simulink model "DaoBaoTin_20151230_Cau2e"  (R2018a)
settings: Solver=FixedStepAuto  StartTime=0.0  StopTime=4  FixedStep=0.01  RelTol=1e-3
values from neighbouring files (symbols this model uses):
  A = [0 1; -0.1 -0.1]    [DaoBaoTin_20151230_Cau1d.m]    (also in DaoBaoTin_20151230_Cau2d.m = [-8.3164 0.0358; -0.7814 -4.0012])
  B = [0.1; 0.09]    [DaoBaoTin_20151230_Cau1d.m]    (also in DaoBaoTin_20151230_Cau2d.m = [0; 2])
  C = [1 0; 0 1]    [DaoBaoTin_20151230_Cau1d.m]    (also in DaoBaoTin_20151230_Cau2d.m)
  D = [0; 0]    [DaoBaoTin_20151230_Cau1d.m]    (also in DaoBaoTin_20151230_Cau2d.m)
  K = H * inv(W)    [DaoBaoTin_20151230_Cau1d.m]    (also in DaoBaoTin_20151230_Cau2d.m)
settings Model: Creator=20151  LastModifiedBy=20151
settings DataIOCC: ReturnWorkspaceOutputs=on
settings DebuggingCC: UnconnectedInputMsg=none  UnconnectedOutputMsg=none  UnconnectedLineMsg=none  SFMachineParentedDataDiag=error
settings SFSimCC: SimUseLocalCustomCode=on
settings RTWCC: RTWUseLocalCustomCode=on

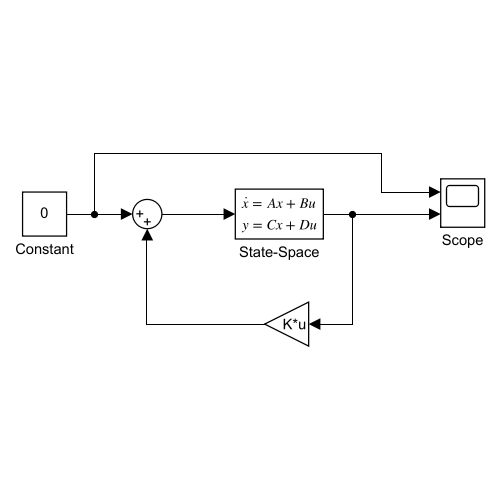
[thumbnail: Simulink's stored preview of the top-level diagram]
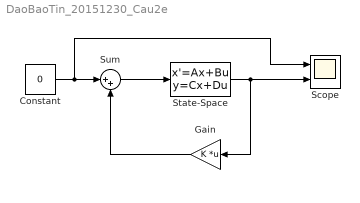
== system DaoBaoTin_20151230_Cau2e ==
  Constant : Constant  Value=0  SampleTime=0.01
  Gain : Gain  Gain=K  Multiplication=Matrix(K*u)
  Scope : Scope  NumInputPorts=2
  State-Space : StateSpace  A=A  B=B  C=C  D=D  InitialCondition=[4 0.2]
  Sum : Sum  Inputs=|++
  wires:
  State-Space/1 -> Gain/1, Scope/2
  Constant/1 -> Sum/1, Scope/1
  Gain/1 -> Sum/2
  Sum/1 -> State-Space/1
